simulink model "ARDroneTTSim_2019"  (Simulink 9.3)
settings: Solver=ode1  StartTime=0.0  StopTime=200  FixedStep=simDT  RelTol=1e-3  EnableMultiTasking=on
values from neighbouring files (symbols this model uses):
  choice = input('')    [setupTTSim.m]
  K = lqr(A,B,Q1,R)    [LOS_Study.m]    (also in setupTTSim.m = lqr(A,B,Q,R))
  k_w = 1    [LOS_Study.m]    (also in setupTTSim.m)
  timeDelay = FMS.Ts*4    [LOS_Study.m]    (also in setupTTSim.m)
undefined symbols (not defined in the file or in its folder): DiscIntNeverNeededParam, FMS, ssH, ssPitch, ssPitch2U, ssRoll, ssRoll2V, ssYaw
libraries: simulink x1, ARBlocks x1
settings Model: Creator=Paul Freeman  LastModifiedBy=User
settings DataIOCC: SaveFormat=Dataset  SignalLogging=off  ReturnWorkspaceOutputs=on
settings OptimizationCC: ExpressionDepthLimit=2147483647
settings DebuggingCC: SolverPrmCheckMsg=warning  MultiTaskDSMMsg=warning  MultiTaskCondExecSysMsg=none  AllowSymbolicDim=off  StateNameClashWarn=warning
settings HardwareCC: ProdLargestAtomicInteger=Long  ProdLargestAtomicFloat=Double  ProdIntDivRoundTo=Zero  ProdEndianess=BigEndian  ProdHWDeviceType=Freescale->32-bit PowerPC
settings SFSimCC: SimParseCustomCode=off
settings ConfigComp: CovHtmlReporting=off

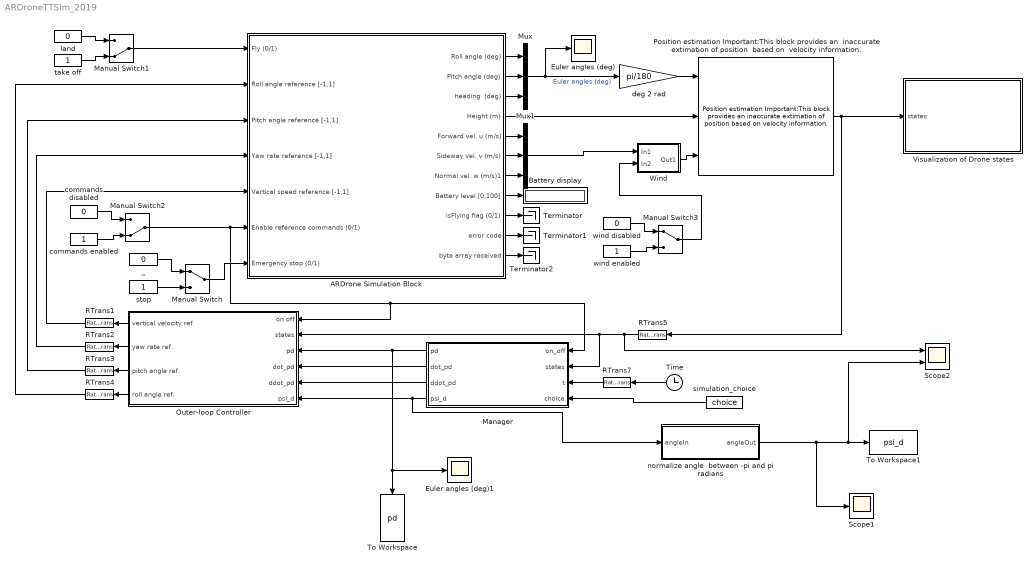
== system ARDroneTTSim_2019 ==
  ARDrone Simulation Block : Subsystem  AncestorBlock=ARBlocks/ARDrone Simulation Block
  Battery display : Display
  Euler angles (deg) : Scope
  Euler angles (deg)1 : Scope
  Manager : MATLAB Function  TreatAsAtomicUnit=on  SystemSampleTime=FMS.Ts
  Manual Switch : ManualSwitch
  Manual Switch1 : ManualSwitch  CurrentSetting=0
  Manual Switch2 : ManualSwitch  CurrentSetting=0
  Manual Switch3 : ManualSwitch
  Mux : Mux  Inputs=3
  Mux1 : Mux  Inputs=3
  Outer-loop Controller : Subsystem
  "Position estimation Important:This block provides an  inaccurate extimation of position  based on  velocity information. " : ARBlocks/Position estimation Important:This block provides an  inaccurate extimation of position  based on  velocity information.   SystemSampleTime=-1
  RTrans{1..4} (4 alike) : RateTransition  OutPortSampleTime=simDT
  RTrans5 : RateTransition  OutPortSampleTime=FMS.Ts
  RTrans7 : RateTransition  OutPortSampleTime=FMS.Ts
  Scope1 : Scope
  Scope2 : Scope  NumInputPorts=2
  Terminator : Terminator
  Terminator1 : Terminator
  Terminator2 : Terminator
  Time : Clock
  To Workspace : ToWorkspace  VariableName=pd  SaveFormat=Structure With Time  SampleTime=-1
  To Workspace1 : ToWorkspace  VariableName=psi_d  SaveFormat=Structure With Time  SampleTime=-1
  Visualization of Drone states : Subsystem
  Wind : Subsystem
  _ : Constant  Value=0
  commands disabled : Constant  Value=0
  commands enabled : Constant
  deg 2 rad : Gain  Gain=pi/180
  land : Constant  Value=0
  normalize angle  between -pi and pi radians : MATLAB Function  TreatAsAtomicUnit=on
  simulation_choice : Constant  Value=choice
  stop : Constant
  take off : Constant
  wind disabled : Constant  Value=0
  wind enabled : Constant
  wires:
  _/1 -> Manual Switch/1
  stop/1 -> Manual Switch/2
  land/1 -> Manual Switch1/1
  take off/1 -> Manual Switch1/2
  commands disabled/1 -> Manual Switch2/1
  commands enabled/1 -> Manual Switch2/2
  Manual Switch1/1 -> ARDrone Simulation Block/1(Fly (0/1))
  Manual Switch/1 -> ARDrone Simulation Block/7(Emergency stop (0/1))
  ARDrone Simulation Block/1(Roll angle (deg)) -> Mux/1
  ARDrone Simulation Block/2(Pitch angle (deg)) -> Mux/2
  ARDrone Simulation Block/5(Forward vel. u (m/s)) -> Mux1/1
  ARDrone Simulation Block/6(Sideway vel. v (m/s)) -> Mux1/2
  ARDrone Simulation Block/7(Normal vel. w (m/s)1) -> Mux1/3
  Mux/1 -> deg 2 rad/1, Euler angles (deg)/1  "Euler angles (deg)"
  ARDrone Simulation Block/8(Battery level [0,100]) -> Battery display/1
  "Position estimation Important:This block provides an  inaccurate extimation of position  based on  velocity information. "/1 -> RTrans5/1, Visualization of Drone states/1(states)
  deg 2 rad/1 -> "Position estimation Important:This block provides an  inaccurate extimation of position  based on  velocity information. "/1
  ARDrone Simulation Block/4(Height (m)) -> "Position estimation Important:This block provides an  inaccurate extimation of position  based on  velocity information. "/2
  Time/1 -> RTrans7/1
  ARDrone Simulation Block/3(heading  (deg)) -> Mux/3
  ARDrone Simulation Block/9(isFlying flag (0/1)) -> Terminator/1
  RTrans1/1 -> ARDrone Simulation Block/5(Vertical speed reference [-1,1])
  RTrans3/1 -> ARDrone Simulation Block/3(Pitch angle reference [-1,1])
  RTrans4/1 -> ARDrone Simulation Block/2(Roll angle reference [-1,1])
  RTrans7/1 -> Manager/3(t)
  ARDrone Simulation Block/10(error code) -> Terminator1/1
  ARDrone Simulation Block/11(byte array received) -> Terminator2/1
  RTrans2/1 -> ARDrone Simulation Block/4(Yaw rate reference [-1,1])
  Manual Switch2/1 -> Manager/1(on_off), Outer-loop Controller/1(on off), ARDrone Simulation Block/6(Enable reference commands (0/1))
  RTrans5/1 -> Scope2/1, Manager/2(states), Outer-loop Controller/2(states)
  Manager/1(pd) -> Euler angles (deg)1/1, To Workspace/1, Outer-loop Controller/3(pd)
  Manager/2(dot_pd) -> Outer-loop Controller/4(dot_pd)
  Manager/3(ddot_pd) -> Outer-loop Controller/5(ddot_pd)
  Manager/4(psi_d) -> normalize angle  between -pi and pi radians/1(angleIn), Outer-loop Controller/6(psi_d)
  Outer-loop Controller/1(vertical velocity ref.) -> RTrans1/1
  Outer-loop Controller/2(yaw rate ref.) -> RTrans2/1
  Outer-loop Controller/3(pitch angle ref.) -> RTrans3/1
  Outer-loop Controller/4(roll angle ref.) -> RTrans4/1
  simulation_choice/1 -> Manager/4(choice)
  normalize angle  between -pi and pi radians/1(angleOut) -> Scope1/1, Scope2/2, To Workspace1/1
  Mux1/1 -> Wind/1(In1)
  Wind/1(Out1) -> "Position estimation Important:This block provides an  inaccurate extimation of position  based on  velocity information. "/3
  wind enabled/1 -> Manual Switch3/2
  wind disabled/1 -> Manual Switch3/1
  Manual Switch3/1 -> Wind/2(In2)

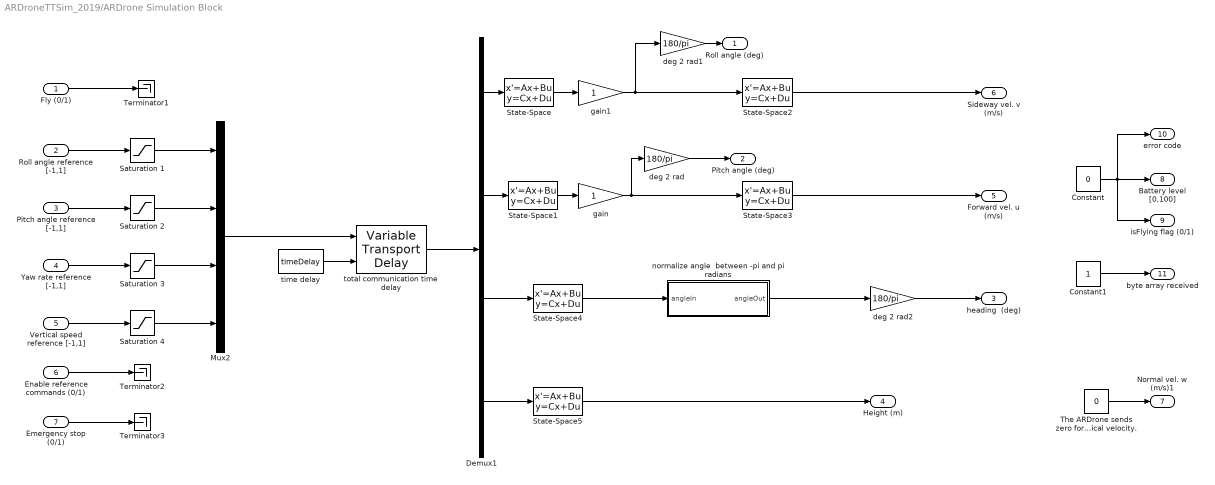
== system ARDroneTTSim_2019/ARDrone Simulation Block ==
  Fly (0/1) : Inport
  Roll angle reference [-1,1] : Inport  Port=2
  Pitch angle reference [-1,1] : Inport  Port=3
  Yaw rate reference [-1,1] : Inport  Port=4
  Vertical speed reference [-1,1] : Inport  Port=5
  Enable reference commands (0/1) : Inport  Port=6
  Emergency stop (0/1) : Inport  Port=7
  Constant : Constant  Value=0
  Constant1 : Constant
  Demux1 : Demux  Outputs=[1,1,1,1]
  Mux2 : Mux  Inputs=[1,1,1,1]
  Saturation {1..4} (4 alike) : Saturate  UpperLimit=1  LowerLimit=-1
  State-Space : StateSpace  A=ssRoll.a  B=ssRoll.b  C=ssRoll.c  D=ssRoll.d  InitialCondition=0
  State-Space1 : StateSpace  A=ssPitch.a  B=ssPitch.b  C=ssPitch.c  D=ssPitch.d  InitialCondition=0
  State-Space2 : StateSpace  A=ssRoll2V.a  B=ssRoll2V.b  C=ssRoll2V.c  D=ssRoll2V.d  InitialCondition=0
  State-Space3 : StateSpace  A=ssPitch2U.a  B=ssPitch2U.b  C=ssPitch2U.c  D=ssPitch2U.d  InitialCondition=0
  State-Space4 : StateSpace  A=ssYaw.a  B=ssYaw.b  C=ssYaw.c  D=ssYaw.d  InitialCondition=pi/4
  State-Space5 : StateSpace  A=ssH.a  B=ssH.b  C=ssH.c  D=ssH.d  InitialCondition=0
  Terminator1 : Terminator
  Terminator2 : Terminator
  Terminator3 : Terminator
  "The ARDrone sends zero for the vertical velocity.  " : Constant  Value=0
  deg 2 rad : Gain  Gain=180/pi
  deg 2 rad1 : Gain  Gain=180/pi
  deg 2 rad2 : Gain  Gain=180/pi
  gain : Gain
  gain1 : Gain
  normalize angle  between -pi and pi radians : MATLAB Function  TreatAsAtomicUnit=on
  time delay : Constant  Value=timeDelay
  total communication time delay : VariableTransportDelay  MaximumDelay=10  InitialOutput=[0 0 0 0]  MaximumPoints=4096
  Roll angle (deg) : Outport
  Pitch angle (deg) : Outport  Port=2
  heading  (deg) : Outport  Port=3
  Height (m) : Outport  Port=4
  Forward vel. u (m/s) : Outport  Port=5
  Sideway vel. v (m/s) : Outport  Port=6
  Normal vel. w (m/s)1 : Outport  Port=7
  Battery level [0,100] : Outport  Port=8
  isFlying flag (0/1) : Outport  Port=9
  error code : Outport  Port=10
  byte array received : Outport  Port=11
  wires:
  "The ARDrone sends zero for the vertical velocity.  "/1 -> Normal vel. w (m/s)1/1
  Constant1/1 -> byte array received/1
  deg 2 rad2/1 -> heading  (deg)/1
  deg 2 rad1/1 -> Roll angle (deg)/1
  deg 2 rad/1 -> Pitch angle (deg)/1
  Constant/1 -> Battery level [0,100]/1, error code/1, isFlying flag (0/1)/1
  State-Space4/1 -> normalize angle  between -pi and pi radians/1(angleIn)
  State-Space5/1 -> Height (m)/1
  Emergency stop (0/1)/1 -> Terminator3/1
  Enable reference commands (0/1)/1 -> Terminator2/1
  Fly (0/1)/1 -> Terminator1/1
  Demux1/3 -> State-Space4/1
  Demux1/2 -> State-Space1/1
  Saturation 4/1 -> Mux2/4
  Saturation 3/1 -> Mux2/3
  Saturation 2/1 -> Mux2/2
  Saturation 1/1 -> Mux2/1
  total communication time delay/1 -> Demux1/1
  Mux2/1 -> total communication time delay/1
  time delay/1 -> total communication time delay/2
  State-Space1/1 -> gain/1
  State-Space/1 -> gain1/1
  Demux1/4 -> State-Space5/1
  Demux1/1 -> State-Space/1
  Vertical speed reference [-1,1]/1 -> Saturation 4/1
  Yaw rate reference [-1,1]/1 -> Saturation 3/1
  Pitch angle reference [-1,1]/1 -> Saturation 2/1
  Roll angle reference [-1,1]/1 -> Saturation 1/1
  gain/1 -> State-Space3/1, deg 2 rad/1
  gain1/1 -> State-Space2/1, deg 2 rad1/1
  State-Space2/1 -> Sideway vel. v (m/s)/1
  State-Space3/1 -> Forward vel. u (m/s)/1
  normalize angle  between -pi and pi radians/1(angleOut) -> deg 2 rad2/1

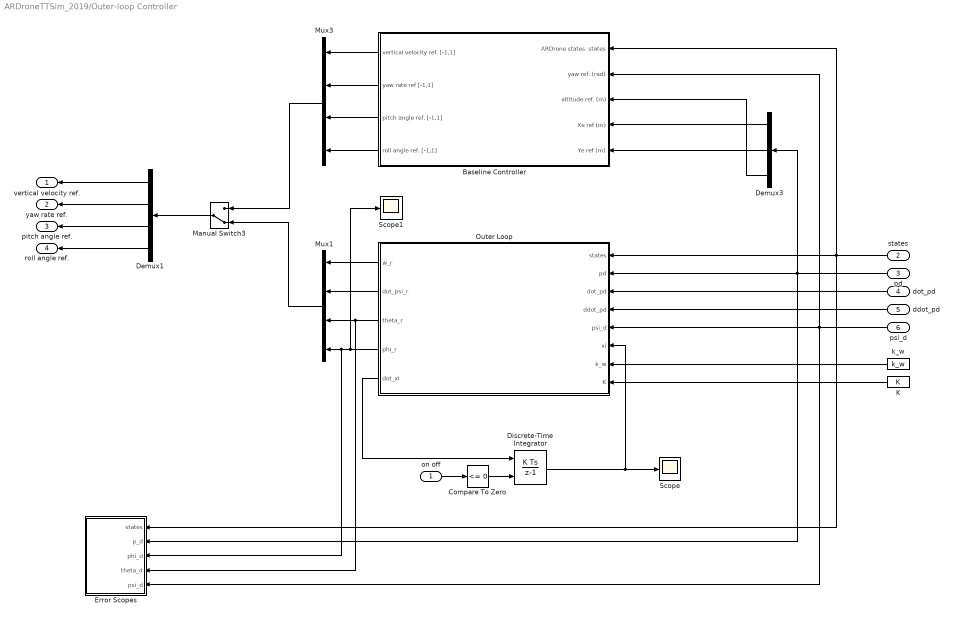
== system ARDroneTTSim_2019/Outer-loop Controller ==
  on off : Inport  PortDimensions=1
  states : Inport  Port=2
  pd : Inport  Port=3  PortDimensions=[3 1]
  dot_pd : Inport  Port=4  PortDimensions=[3 1]
  ddot_pd : Inport  Port=5  PortDimensions=[3 1]
  psi_d : Inport  Port=6  PortDimensions=1
  Baseline Controller : Subsystem  AncestorBlock=ARBlocks/Baseline Controller
  Compare To Zero : simulink/Logic and Bit Operations/Compare To Zero  relop=<=  OutDataTypeStr=boolean
  Demux1 : Demux  Outputs=[1,1,1,1]
  Demux3 : Demux  Outputs=[1,1,1]
  Discrete-Time Integrator : DiscreteIntegrator  ExternalReset=level  InitialCondition=[0;0;0;0]  SampleTime=FMS.Ts  UpperSaturationLimit=10  LowerSaturationLimit=-10  ICPrevOutput=DiscIntNeverNeededParam  ICPrevScaledInput=DiscIntNeverNeededParam
  Error Scopes : Subsystem
  K : Constant  Value=K
  Manual Switch3 : ManualSwitch  CurrentSetting=0
  Mux1 : Mux  Inputs=[1,1,1,1]
  Mux3 : Mux  Inputs=[1,1,1,1]
  Outer Loop : MATLAB Function  TreatAsAtomicUnit=on  SystemSampleTime=FMS.Ts
  Scope : Scope
  Scope1 : Scope
  k_w : Constant  Value=k_w
  vertical velocity ref. : Outport
  yaw rate ref. : Outport  Port=2
  pitch angle ref. : Outport  Port=3
  roll angle ref. : Outport  Port=4
  wires:
  states/1 -> Error Scopes/1(states), Baseline Controller/1("ARDrone states  states "), Outer Loop/1(states)
  Outer Loop/5(dot_xi) -> Discrete-Time Integrator/1
  pd/1 -> Outer Loop/2(pd), Error Scopes/2(p_d), Demux3/1
  dot_pd/1 -> Outer Loop/3(dot_pd)
  ddot_pd/1 -> Outer Loop/4(ddot_pd)
  Demux3/1 -> Baseline Controller/4(Xe ref (m))
  Demux3/2 -> Baseline Controller/5(Ye ref (m))
  Demux3/3 -> Baseline Controller/3(altitude ref. (m))
  Baseline Controller/4(roll angle ref. [-1,1]) -> Mux3/4
  Baseline Controller/3(pitch angle ref. [-1,1]) -> Mux3/3
  Baseline Controller/2(yaw rate ref [-1,1]) -> Mux3/2
  Baseline Controller/1(vertical velocity ref. [-1,1]) -> Mux3/1
  Mux3/1 -> Manual Switch3/1
  Demux1/1 -> vertical velocity ref./1
  Demux1/2 -> yaw rate ref./1
  Demux1/3 -> pitch angle ref./1
  Demux1/4 -> roll angle ref./1
  Manual Switch3/1 -> Demux1/1
  Mux1/1 -> Manual Switch3/2
  on off/1 -> Compare To Zero/1
  Compare To Zero/1 -> Discrete-Time Integrator/2
  k_w/1 -> Outer Loop/7(k_w)
  K/1 -> Outer Loop/8(K)
  Outer Loop/1(w_r) -> Mux1/1
  Outer Loop/2(dot_psi_r) -> Mux1/2
  Outer Loop/3(theta_r) -> Error Scopes/4(theta_d), Mux1/3
  Outer Loop/4(phi_r) -> Scope1/1, Mux1/4, Error Scopes/3(phi_d)
  Discrete-Time Integrator/1 -> Outer Loop/6(xi), Scope/1
  psi_d/1 -> Error Scopes/5(psi_d), Outer Loop/5(psi_d), Baseline Controller/2(yaw ref. (rad))

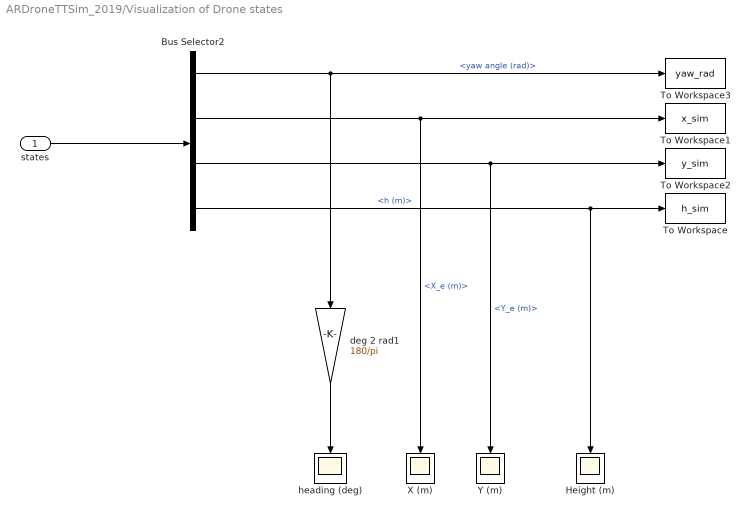
== system ARDroneTTSim_2019/Visualization of Drone states ==
  states : Inport
  Bus Selector2 : BusSelector  OutputSignals=yaw angle (rad),X_e (m),Y_e (m),h (m)
  Height (m) : Scope
  To Workspace : ToWorkspace  VariableName=h_sim  SaveFormat=Structure With Time  SampleTime=-1
  To Workspace1 : ToWorkspace  VariableName=x_sim  SaveFormat=Structure With Time  SampleTime=-1
  To Workspace2 : ToWorkspace  VariableName=y_sim  SaveFormat=Structure With Time  SampleTime=-1
  To Workspace3 : ToWorkspace  VariableName=yaw_rad  SaveFormat=Structure With Time  SampleTime=-1
  X (m) : Scope
  Y (m) : Scope
  deg 2 rad1 : Gain  Gain=180/pi
  heading (deg) : Scope
  wires:
  states/1 -> Bus Selector2/1
  Bus Selector2/1 -> To Workspace3/1, deg 2 rad1/1  "<yaw angle (rad)>"
  Bus Selector2/2 -> X (m)/1, To Workspace1/1  "<X_e (m)>"
  Bus Selector2/3 -> To Workspace2/1, Y (m)/1  "<Y_e (m)>"
  Bus Selector2/4 -> Height (m)/1, To Workspace/1  "<h (m)>"
  deg 2 rad1/1 -> heading (deg)/1

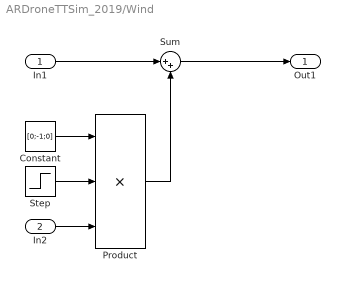
== system ARDroneTTSim_2019/Wind ==
  In1 : Inport
  In2 : Inport  Port=2
  Constant : Constant  Value=[0;-1;0]
  Product : Product  Inputs=3
  Step : Step  Time=20  SampleTime=0
  Sum : Sum  Inputs=|++
  Out1 : Outport
  wires:
  Sum/1 -> Out1/1
  In1/1 -> Sum/1
  Product/1 -> Sum/2
  Step/1 -> Product/2
  Constant/1 -> Product/1
  In2/1 -> Product/3

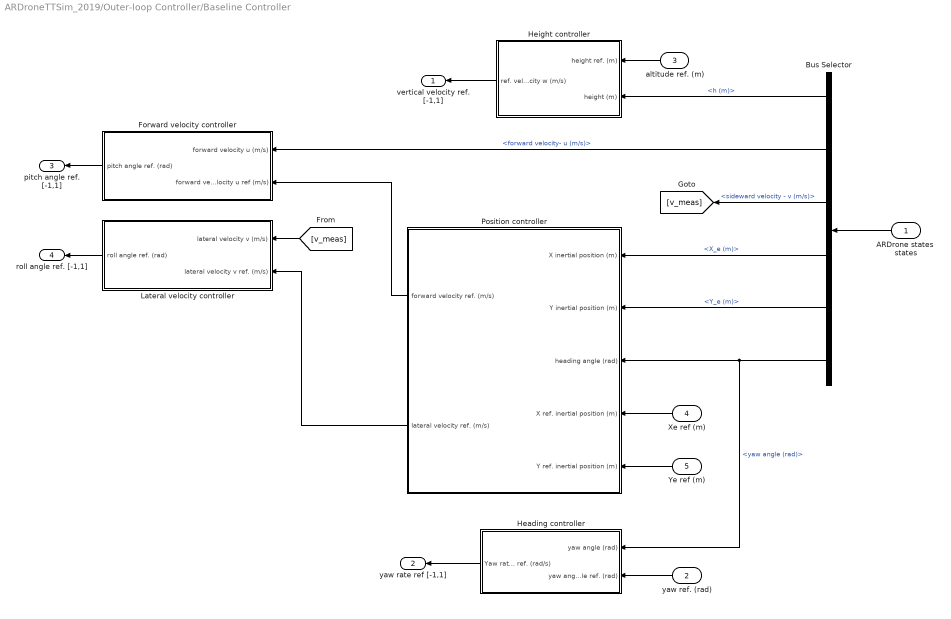
== system ARDroneTTSim_2019/Outer-loop Controller/Baseline Controller ==
  "ARDrone states  states " : Inport
  yaw ref. (rad) : Inport  Port=2
  altitude ref. (m) : Inport  Port=3
  Xe ref (m) : Inport  Port=4
  Ye ref (m) : Inport  Port=5
  Bus Selector : BusSelector  OutputSignals=h (m),forward velocity- u (m/s),sideward velocity - v (m/s),X_e (m),Y_e (m),yaw angle (rad)
  "Forward velocity controller " : Subsystem
  Heading controller : Subsystem
  "Height controller " : Subsystem
  Lateral velocity controller : Subsystem
  Position controller : Subsystem
  vertical velocity ref. [-1,1] : Outport
  yaw rate ref [-1,1] : Outport  Port=2
  pitch angle ref. [-1,1] : Outport  Port=3
  roll angle ref. [-1,1] : Outport  Port=4
  wires:
  [v_meas] -> Lateral velocity controller/1(lateral velocity v (m/s))
  Bus Selector/3 -> [v_meas]  "<sideward velocity - v (m/s)>"
  Position controller/2(lateral velocity ref. (m/s)) -> Lateral velocity controller/2(lateral velocity v ref. (m/s))
  Position controller/1(forward velocity ref. (m/s)) -> "Forward velocity controller "/2(forward velocity u ref (m/s))
  Ye ref (m)/1 -> Position controller/5(Y ref. inertial position (m))
  Xe ref (m)/1 -> Position controller/4(X ref. inertial position (m))
  Bus Selector/5 -> Position controller/2(Y inertial position (m))  "<Y_e (m)>"
  Bus Selector/4 -> Position controller/1(X inertial position (m))  "<X_e (m)>"
  Heading controller/1(Yaw rate ref. (rad/s)) -> yaw rate ref [-1,1]/1
  yaw ref. (rad)/1 -> Heading controller/2(yaw angle ref. (rad))
  "Forward velocity controller "/1(pitch angle ref. (rad)) -> pitch angle ref. [-1,1]/1
  Bus Selector/2 -> "Forward velocity controller "/1(forward velocity u (m/s))  "<forward velocity- u (m/s)>"
  Lateral velocity controller/1(roll angle ref. (rad)) -> roll angle ref. [-1,1]/1
  "Height controller "/1(ref. velocity w (m/s)) -> vertical velocity ref. [-1,1]/1
  Bus Selector/1 -> "Height controller "/2(height (m))  "<h (m)>"
  altitude ref. (m)/1 -> "Height controller "/1(height ref. (m))
  "ARDrone states  states "/1 -> Bus Selector/1
  Bus Selector/6 -> Position controller/3(heading angle (rad)), Heading controller/1(yaw angle (rad))  "<yaw angle (rad)>"

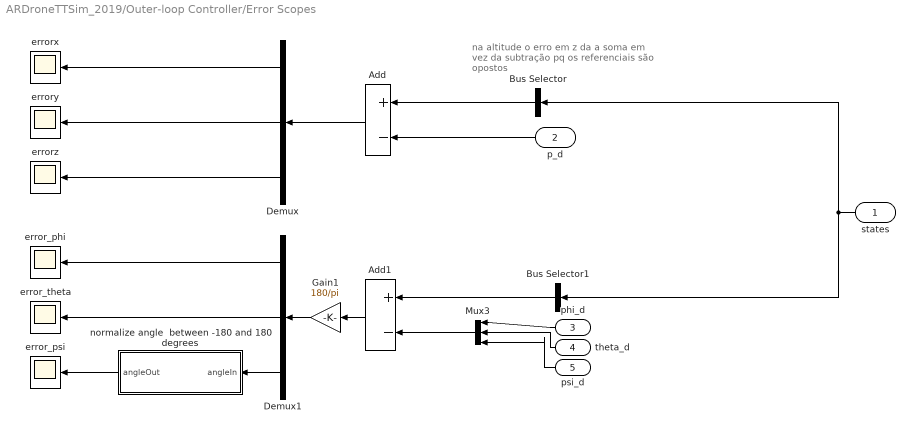
== system ARDroneTTSim_2019/Outer-loop Controller/Error Scopes ==
  note: na altitude o erro em z da a soma em vez da subtração pq os referenciais são opostos
  states : Inport
  p_d : Inport  Port=2
  phi_d : Inport  Port=3
  theta_d : Inport  Port=4
  psi_d : Inport  Port=5
  Add : Sum  Inputs=+-
  Add1 : Sum  Inputs=+-
  Bus Selector : BusSelector  OutputSignals=X_e (m),Y_e (m),h (m)  OutputAsBus=on
  Bus Selector1 : BusSelector  OutputSignals=roll angle (rad),pitch angle (rad),yaw angle (rad)  OutputAsBus=on
  Demux : Demux  Outputs=3
  Demux1 : Demux  Outputs=3
  Gain1 : Gain  Gain=180/pi
  Mux3 : Mux  Inputs=[1,1,1]
  error_phi : Scope
  error_psi : Scope
  error_theta : Scope
  errorx : Scope
  errory : Scope
  errorz : Scope
  normalize angle  between -180 and 180 degrees : MATLAB Function  TreatAsAtomicUnit=on
  wires:
  Demux/1 -> errorx/1
  Demux/3 -> errorz/1
  Demux/2 -> errory/1
  phi_d/1 -> Mux3/1
  theta_d/1 -> Mux3/2
  psi_d/1 -> Mux3/3
  states/1 -> Bus Selector/1, Bus Selector1/1
  Add1/1 -> Gain1/1
  Demux1/3 -> normalize angle  between -180 and 180 degrees/1(angleIn)
  Demux1/2 -> error_theta/1
  p_d/1 -> Add/2
  Add/1 -> Demux/1
  Bus Selector/1 -> Add/1
  Mux3/1 -> Add1/2
  Bus Selector1/1 -> Add1/1
  Demux1/1 -> error_phi/1
  Gain1/1 -> Demux1/1
  normalize angle  between -180 and 180 degrees/1(angleOut) -> error_psi/1

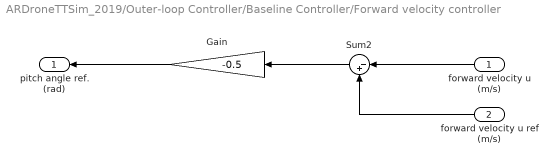
== system ARDroneTTSim_2019/Outer-loop Controller/Baseline Controller/Forward velocity controller  ==
  forward velocity u (m/s) : Inport
  forward velocity u ref (m/s) : Inport  Port=2
  Gain : Gain  Gain=-0.5
  Sum2 : Sum  Inputs=|-+
  pitch angle ref. (rad) : Outport
  wires:
  forward velocity u ref (m/s)/1 -> Sum2/2
  Gain/1 -> pitch angle ref. (rad)/1
  Sum2/1 -> Gain/1
  forward velocity u (m/s)/1 -> Sum2/1

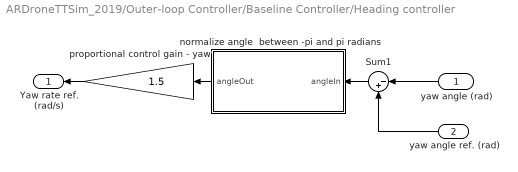
== system ARDroneTTSim_2019/Outer-loop Controller/Baseline Controller/Heading controller ==
  yaw angle (rad) : Inport
  yaw angle ref. (rad) : Inport  Port=2
  Sum1 : Sum  Inputs=|-+
  normalize angle  between -pi and pi radians : MATLAB Function  TreatAsAtomicUnit=on
  proportional control gain - yaw : Gain  Gain=1.5
  Yaw rate ref. (rad/s) : Outport
  wires:
  yaw angle ref. (rad)/1 -> Sum1/2
  proportional control gain - yaw/1 -> Yaw rate ref. (rad/s)/1
  yaw angle (rad)/1 -> Sum1/1
  normalize angle  between -pi and pi radians/1(angleOut) -> proportional control gain - yaw/1
  Sum1/1 -> normalize angle  between -pi and pi radians/1(angleIn)

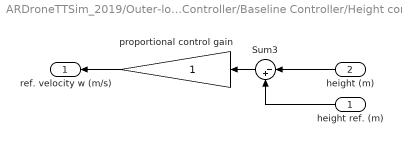
== system ARDroneTTSim_2019/Outer-loop Controller/Baseline Controller/Height controller  ==
  height ref. (m) : Inport
  height (m) : Inport  Port=2
  Sum3 : Sum  Inputs=|-+
  proportional control gain : Gain
  ref. velocity w (m/s) : Outport
  wires:
  height ref. (m)/1 -> Sum3/2
  height (m)/1 -> Sum3/1
  Sum3/1 -> proportional control gain/1
  proportional control gain/1 -> ref. velocity w (m/s)/1

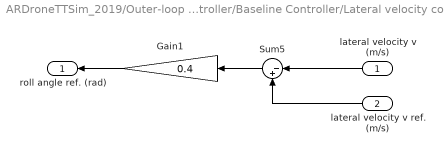
== system ARDroneTTSim_2019/Outer-loop Controller/Baseline Controller/Lateral velocity controller ==
  lateral velocity v (m/s) : Inport
  lateral velocity v ref. (m/s) : Inport  Port=2
  Gain1 : Gain  Gain=0.4
  Sum5 : Sum  Inputs=|-+
  roll angle ref. (rad) : Outport
  wires:
  lateral velocity v ref. (m/s)/1 -> Sum5/2
  Gain1/1 -> roll angle ref. (rad)/1
  Sum5/1 -> Gain1/1
  lateral velocity v (m/s)/1 -> Sum5/1

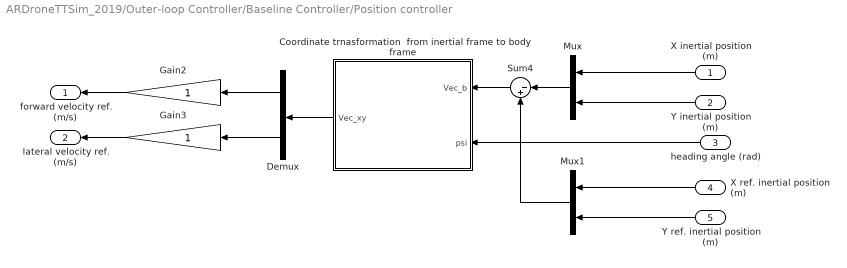
== system ARDroneTTSim_2019/Outer-loop Controller/Baseline Controller/Position controller ==
  X inertial position (m) : Inport
  Y inertial position (m) : Inport  Port=2
  heading angle (rad) : Inport  Port=3
  X ref. inertial position (m) : Inport  Port=4
  Y ref. inertial position (m) : Inport  Port=5
  "Coordinate trnasformation  from inertial frame to body frame " : MATLAB Function  TreatAsAtomicUnit=on
  Demux : Demux  Outputs=2
  Gain2 : Gain
  Gain3 : Gain
  Mux : Mux  Inputs=2
  Mux1 : Mux  Inputs=2
  Sum4 : Sum  Inputs=|-+
  forward velocity ref. (m/s) : Outport
  lateral velocity ref. (m/s) : Outport  Port=2
  wires:
  Gain3/1 -> lateral velocity ref. (m/s)/1
  Demux/2 -> Gain3/1
  Demux/1 -> Gain2/1
  Y ref. inertial position (m)/1 -> Mux1/2
  X ref. inertial position (m)/1 -> Mux1/1
  Mux/1 -> Sum4/1
  X inertial position (m)/1 -> Mux/1
  Y inertial position (m)/1 -> Mux/2
  Sum4/1 -> "Coordinate trnasformation  from inertial frame to body frame "/1(Vec_b)
  Mux1/1 -> Sum4/2
  "Coordinate trnasformation  from inertial frame to body frame "/1(Vec_xy) -> Demux/1
  heading angle (rad)/1 -> "Coordinate trnasformation  from inertial frame to body frame "/2(psi)
  Gain2/1 -> forward velocity ref. (m/s)/1

== matlab function Manager ==
  data: on_off input double; states input double; t input double; pd output double; dot_pd output double; ddot_pd output double; psi_d output double; choice input double
function [pd, dot_pd, ddot_pd, psi_d] = desired_trajectory(on_off,states,t, choice)
%#codegen

% ------------------------------------------------------------------------
% inputs:
% on_off - 1 if tracking is on, 0 if it is off
% states - structure with state variables
% t - current simulation time
% 
% outputs:
% pd - desired position
% dot_pd - desired velocity
% ddot_pd - desired acceleration
% psi_d - desired yaw angle
% ------------------------------------------------------------------------

persistent t0
persistent p0
persistent previous_status

on  = 1;
off = 0;

BASE_ALT = 1;

% RESETS THE 0
if isempty(previous_status)
    previous_status = on;
    p0 = [states(7:8);BASE_ALT];
end

if on_off == off
    if previous_status == on 
    % first time off or switching back off
        p0 = [states(7:8);BASE_ALT]; % x0 and y0 match the current position
    end
    pd = p0;
    dot_pd = [0;0;0];
    ddot_pd = [0;0;0];
    psi_d = 0;
else
    if isempty(t0) || (previous_status == off) 
    % first time on or switching back on
        t0 = t;
        p0 = [states(7:8);BASE_ALT];
    end
    dt = t-t0;

%!!!!!!!!!!!!!!!!!!!!!!!!!!!!!!!!!!!!!!!!!!!!!!!!!!!!!!!!!!!!!!!!!!!!!!!!
% replace with the necessary code to define adequate desired trajectories
% use dt, p0, and any additional parameters

pd      = p0;
t_init  = 10;
t_track = 20;

% DEFINES THE STARTING HEIGHT
if(dt > t_init)
    pd(3) = pd(3) + 0.25;  
else
    pd(3) = pd(3) + 0;  
end

% DIFFERENT TRACKS
switch choice
    %--- Altitude Tracking ---
    case 1
      dot_pd    = [0;0;0];
      ddot_pd   = [0;0;0];
      psi_d     = 0;
    % --- Horizontal Line in X-Y ---
    case 2
      ang = 45;
      vel = 0.1;

      if(dt > t_track)
        dot_pd  = [vel*cosd(ang); vel*sind(ang);0];
        pd(1)   = p0(1) + vel*cosd(ang)*(dt - t_track);
        pd(2)   = p0(2) + vel*sind(ang)*(dt - t_track);
      else
        dot_pd  = [0;0;0]; 
      end
      
      ddot_pd   = [0;0;0];
      psi_d     = 0;
    % --- Circular Line - Constant Yaw ---
	case 3
      ang_rate = 0.1; %rad/s

      if(dt > t_track)
        pd(1:2)	= [ cos(ang_rate*(dt - t_track)) - 1;... 
                    sin(ang_rate*(dt - t_track))];
        dot_pd	= [-sin(ang_rate*(dt - t_track));...
                    cos(ang_rate*(dt - t_track));0]*ang_rate;
        ddot_pd = [-cos(ang_rate*(dt - t_track));...
                   -sin(ang_rate*(dt - t_track));0]*(ang_rate^2);
      else
        dot_pd  = [0;0;0]; 
        ddot_pd = [0;0;0]; 
      end
      psi_d = 0;
    % --- Circular Line - Variable Yaw ---
    case 4
      ang_rate  = 0.1; %rad/s
      R         = 1;
      if(dt > t_track)
        pd(1:2)	= [ cos(ang_rate*(dt - t_track)) - 1;... 
                    sin(ang_rate*(dt - t_track))  ]*R;
        dot_pd	= [-sin(ang_rate*(dt - t_track));...
                    cos(ang_rate*(dt - t_track));0]*R*ang_rate;
        ddot_pd = [-cos(ang_rate*(dt - t_track));...
                   -sin(ang_rate*(dt - t_track));0]*R*(ang_rate^2);
        %psi_d = pi/2;
        psi_d   =       ang_rate*(dt - t_track);
      else
        dot_pd  = [0;0;0]; 
        ddot_pd = [0;0;0];
        psi_d   = 0;
      end
    % --- Line of Sight ---
    case 5
      Delta  = 0.3; 
      V      = 0.1;
      yd     = p0(2) + 1;
      %vel = 0.1;
      if(dt > t_track)
        %pd(1:2)	= p0(1:2) + [V*(dt - t_track); 1];
        pd(1:2)   = states(7:8);
        psi_d     = atan(-(states(8) - yd)/Delta);
        dot_pd	  = [cos(psi_d);sin(psi_d);0]*V;
        %ddot_pd   = [0;0;0];
        dot_psi_d = (-states(5)/Delta)/(1+(-(states(8)-yd)/Delta)^2);
        ddot_pd   = [-V*dot_psi_d*sin(psi_d); V*dot_psi_d*cos(psi_d); 0];
      else
        dot_pd  = [0;0;0]; 
        ddot_pd = [0;0;0];
        psi_d   = 0;
      end  
    otherwise
      pd        = p0;
      dot_pd    = [0;0;0];
      ddot_pd   = [0;0;0];
      psi_d     = 0;
end
        
%!!!!!!!!!!!!!!!!!!!!!!!!!!!!!!!!!!!!!!!!!!!!!!!!!!!!!!!!!!!!!!!!!!!!!!!!

end

previous_status = on_off;

== matlab function Outer-loop Controller/Outer Loop ==
  data: w_r output double; dot_psi_r output double; theta_r output double; states input double; pd input double; dot_pd input double; ddot_pd input double; psi_d input double; xi input double; phi_r output double; dot_xi output double; k_w input double; K input double
function [w_r, dot_psi_r, theta_r, phi_r, dot_xi] = tt_controller(states, pd, dot_pd, ddot_pd,psi_d,xi, k_w, K)
%#codegen

% ------------------------------------------------------------------------
% inputs:
% states - structure with state variables
% pd - desired position
% dot_pd - desired velocity
% ddot_pt - desired acceleration
% psi_d - desired yaw angle
% xi - integral state (four variables)
%
% outputs:
% w_r - vertical velocity reference
% dot_psi_r - yaw rate reference
% theta_r - pitch angle reference
% phi_r - roll angle reference
% dot_xi - integral state derivative
% ------------------------------------------------------------------------

lambda      = states(1:3,1); % Euler angles
psi         = lambda(3);
R           = euler2R(lambda);
Rz          = [cos(psi) -sin(psi) 0; sin(psi) cos(psi) 0; 0 0 1];
psi_e       = normalize_angle(psi-psi_d);

p           = states(7:9,1); % position vector
p(3)        = p(3); % height is symmetric of z
vb          = states(4:6,1); % velocity vector in body coordinates
dot_p       = R*vb; % body velocity rotated to inertial frame 
dot_p(3)    = dot_p(3);

%!!!!!!!!!!!!!!!!!!!!!!!!!!!!!!!!!!!!!!!!!!!!!!!!!!!!!!!!!!!!!!!!!!!!!!
% replace with the necessary code to implement the trajectory tracking
% controller
% pd(3)       = pd(3);
% dot_pd(3)   = dot_pd(3);

% HEIGHT CONTROL
w_r     = -k_w*(p(3) - pd(3));

% OTHER CONTROL
tilde_x     = [p - pd; dot_p - dot_pd];

u_star      = Rz^(-1)*(K*tilde_x + [0; 0; 9.81] - ddot_pd + xi(1:3));

theta_r     = atan(u_star(1)/u_star(3));
phi_r       = atan(-u_star(2)/sqrt(u_star(1)^2+u_star(3)^2));
dot_xi      = [k_w*1*K*tilde_x; psi_e];
dot_xi(3)   = dot_xi(3);

% PSI CONTROL
dot_psi_r   = -1*psi_e - 0.1*xi(4);
%!!!!!!!!!!!!!!!!!!!!!!!!!!!!!!!!!!!!!!!!!!!!!!!!!!!!!!!!!!!!!!!!!!!!!!


function R = euler2R(l)
%#codegen
% returns the rotation matrix for a given vector of euler angles

phi = l(1); theta = l(2); psi = l(3);
R = [cos(theta)*cos(psi)...
      sin(phi)*sin(theta)*cos(psi)-cos(phi)*sin(psi)...
      cos(phi)*sin(theta)*cos(psi)+sin(phi)*sin(psi);
   cos(theta)*sin(psi)...
   sin(phi)*sin(theta)*sin(psi)+cos(phi)*cos(psi)... 
   cos(phi)*sin(theta)*sin(psi)-sin(phi)*cos(psi);
   -sin(theta)...
   sin(phi)*cos(theta)...
   cos(phi)*cos(theta)];

function angleOut = normalize_angle(angleIn)
%#codegen

angleOut = mod(angleIn, 2*pi) ;
if angleOut > pi
    angleOut = -2*pi + angleOut ; 
end

== matlab function normalize angle between -pi and pi radians ==
  data: angleIn input double; angleOut output double
function angleOut = fcn(angleIn)
%#codegen

angleOut = mod(angleIn, 2*pi) ;
if angleOut > pi
    angleOut = -2*pi + angleOut ; 
end

== matlab function Outer-loop Controller/Baseline Controller/Heading controller/normalize angle between -pi and pi radians ==
  data: angleIn input double; angleOut output double
function angleOut = fcn(angleIn)
%#codegen

angleOut = mod(angleIn, 2*pi) ;
if angleOut > pi
    angleOut = -2*pi + angleOut ; 
end

== matlab function ARDrone Simulation Block/normalize angle between -pi and pi radians ==
  data: angleIn input double; angleOut output double
function angleOut = fcn(angleIn)
%#codegen

angleOut = mod(angleIn, 2*pi) ;
if angleOut > pi
    angleOut = -2*pi + angleOut ; 
end

== matlab function Outer-loop Controller/Baseline Controller/Position controller/Coordinate trnasformation from inertial frame to body frame  ==
  data: Vec_b input double; Vec_xy output double; psi input double
function Vec_xy  = fcn(Vec_b , psi)
%#codegen
T = [cos(psi) sin(psi) ; -sin(psi) cos(psi)] ; 
Vec_xy = T*Vec_b(1:2,1);

== matlab function Outer-loop Controller/Error Scopes/normalize angle between -180 and 180 degrees ==
  data: angleIn input double; angleOut output double
function angleOut = fcn(angleIn)
%#codegen

angleOut = mod(angleIn, 360) ;
if angleOut > 180
    angleOut = -360 + angleOut ; 
end
